simulink model "snap2_f_200msps_64i_4096c"  (R2019a)
settings: Solver=VariableStepDiscrete  StartTime=0.0  StopTime=10.0  RelTol=1e-3
undefined symbols (not defined in the file or in its folder): datetime, posixtime
libraries: xbsIndex_r4 x21354, casper_library_misc x297, casper_library_delays x19, xps_library x14, casper_library_sources x4
(part 60 of 217)

== system snap2_f_200msps_64i_4096c/delay/Subsystem/2 ==
  din : Inport
  delay : Inport  Port=2
  Slice : xbsIndex_r4/Slice  nbits=10  boolean_output=off  mode=Lower Bit Location + Width  bit1=0  base1=MSB of Input  bit0=0  base0=LSB of Input  dbl_ovrd=off  block_type=slice
  Slice1 : xbsIndex_r4/Slice  nbits=2  boolean_output=off  mode=Lower Bit Location + Width  bit1=0  base1=MSB of Input  bit0=10  base0=LSB of Input  dbl_ovrd=off  block_type=slice
  Subsystem1 : Subsystem
  delay_bram_prog_dp : Subsystem  AncestorBlock=casper_library_delays/delay_bram_prog_dp  mask(delay_bram_prog_dp){ram_bits=max_delay_bits-2, bram_latency=2, async=off}
      mask prompts: ram_bits "Max delay (2^?)"; bram_latency "BRAM latency"; async "asynchronous operation"
      mask init:
      | delay_bram_prog_dp_init(gcb, ...
      |     'ram_bits', ram_bits, ...
      |     'bram_latency', bram_latency, ...
      |     'async', async);
  dout : Outport
  wires:
  din/1 -> delay_bram_prog_dp/1(din)
  delay/1 -> Slice1/1, Slice/1
  Slice/1 -> delay_bram_prog_dp/2(delay)
  Slice1/1 -> Subsystem1/2(delay)
  delay_bram_prog_dp/1(dout) -> Subsystem1/1(din)
  Subsystem1/1(dout) -> dout/1

== system snap2_f_200msps_64i_4096c/delay/Subsystem/20 ==
  din : Inport
  delay : Inport  Port=2
  Slice : xbsIndex_r4/Slice  nbits=10  boolean_output=off  mode=Lower Bit Location + Width  bit1=0  base1=MSB of Input  bit0=0  base0=LSB of Input  dbl_ovrd=off  block_type=slice
  Slice1 : xbsIndex_r4/Slice  nbits=2  boolean_output=off  mode=Lower Bit Location + Width  bit1=0  base1=MSB of Input  bit0=10  base0=LSB of Input  dbl_ovrd=off  block_type=slice
  Subsystem1 : Subsystem
  delay_bram_prog_dp : Subsystem  AncestorBlock=casper_library_delays/delay_bram_prog_dp  mask(delay_bram_prog_dp){ram_bits=max_delay_bits-2, bram_latency=2, async=off}
      mask prompts: ram_bits "Max delay (2^?)"; bram_latency "BRAM latency"; async "asynchronous operation"
      mask init:
      | delay_bram_prog_dp_init(gcb, ...
      |     'ram_bits', ram_bits, ...
      |     'bram_latency', bram_latency, ...
      |     'async', async);
  dout : Outport
  wires:
  Subsystem1/1(dout) -> dout/1
  delay_bram_prog_dp/1(dout) -> Subsystem1/1(din)
  Slice1/1 -> Subsystem1/2(delay)
  Slice/1 -> delay_bram_prog_dp/2(delay)
  delay/1 -> Slice/1, Slice1/1
  din/1 -> delay_bram_prog_dp/1(din)

== system snap2_f_200msps_64i_4096c/delay/Subsystem/21 ==
  din : Inport
  delay : Inport  Port=2
  Slice : xbsIndex_r4/Slice  nbits=10  boolean_output=off  mode=Lower Bit Location + Width  bit1=0  base1=MSB of Input  bit0=0  base0=LSB of Input  dbl_ovrd=off  block_type=slice
  Slice1 : xbsIndex_r4/Slice  nbits=2  boolean_output=off  mode=Lower Bit Location + Width  bit1=0  base1=MSB of Input  bit0=10  base0=LSB of Input  dbl_ovrd=off  block_type=slice
  Subsystem1 : Subsystem
  delay_bram_prog_dp : Subsystem  AncestorBlock=casper_library_delays/delay_bram_prog_dp  mask(delay_bram_prog_dp){ram_bits=max_delay_bits-2, bram_latency=2, async=off}
      mask prompts: ram_bits "Max delay (2^?)"; bram_latency "BRAM latency"; async "asynchronous operation"
      mask init:
      | delay_bram_prog_dp_init(gcb, ...
      |     'ram_bits', ram_bits, ...
      |     'bram_latency', bram_latency, ...
      |     'async', async);
  dout : Outport
  wires:
  din/1 -> delay_bram_prog_dp/1(din)
  delay/1 -> Slice1/1, Slice/1
  Slice/1 -> delay_bram_prog_dp/2(delay)
  Slice1/1 -> Subsystem1/2(delay)
  delay_bram_prog_dp/1(dout) -> Subsystem1/1(din)
  Subsystem1/1(dout) -> dout/1

== system snap2_f_200msps_64i_4096c/delay/Subsystem/22 ==
  din : Inport
  delay : Inport  Port=2
  Slice : xbsIndex_r4/Slice  nbits=10  boolean_output=off  mode=Lower Bit Location + Width  bit1=0  base1=MSB of Input  bit0=0  base0=LSB of Input  dbl_ovrd=off  block_type=slice
  Slice1 : xbsIndex_r4/Slice  nbits=2  boolean_output=off  mode=Lower Bit Location + Width  bit1=0  base1=MSB of Input  bit0=10  base0=LSB of Input  dbl_ovrd=off  block_type=slice
  Subsystem1 : Subsystem
  delay_bram_prog_dp : Subsystem  AncestorBlock=casper_library_delays/delay_bram_prog_dp  mask(delay_bram_prog_dp){ram_bits=max_delay_bits-2, bram_latency=2, async=off}
      mask prompts: ram_bits "Max delay (2^?)"; bram_latency "BRAM latency"; async "asynchronous operation"
      mask init:
      | delay_bram_prog_dp_init(gcb, ...
      |     'ram_bits', ram_bits, ...
      |     'bram_latency', bram_latency, ...
      |     'async', async);
  dout : Outport
  wires:
  Subsystem1/1(dout) -> dout/1
  delay_bram_prog_dp/1(dout) -> Subsystem1/1(din)
  Slice1/1 -> Subsystem1/2(delay)
  Slice/1 -> delay_bram_prog_dp/2(delay)
  delay/1 -> Slice/1, Slice1/1
  din/1 -> delay_bram_prog_dp/1(din)

== system snap2_f_200msps_64i_4096c/delay/Subsystem/23 ==
  din : Inport
  delay : Inport  Port=2
  Slice : xbsIndex_r4/Slice  nbits=10  boolean_output=off  mode=Lower Bit Location + Width  bit1=0  base1=MSB of Input  bit0=0  base0=LSB of Input  dbl_ovrd=off  block_type=slice
  Slice1 : xbsIndex_r4/Slice  nbits=2  boolean_output=off  mode=Lower Bit Location + Width  bit1=0  base1=MSB of Input  bit0=10  base0=LSB of Input  dbl_ovrd=off  block_type=slice
  Subsystem1 : Subsystem
  delay_bram_prog_dp : Subsystem  AncestorBlock=casper_library_delays/delay_bram_prog_dp  mask(delay_bram_prog_dp){ram_bits=max_delay_bits-2, bram_latency=2, async=off}
      mask prompts: ram_bits "Max delay (2^?)"; bram_latency "BRAM latency"; async "asynchronous operation"
      mask init:
      | delay_bram_prog_dp_init(gcb, ...
      |     'ram_bits', ram_bits, ...
      |     'bram_latency', bram_latency, ...
      |     'async', async);
  dout : Outport
  wires:
  din/1 -> delay_bram_prog_dp/1(din)
  delay/1 -> Slice1/1, Slice/1
  Slice/1 -> delay_bram_prog_dp/2(delay)
  Slice1/1 -> Subsystem1/2(delay)
  delay_bram_prog_dp/1(dout) -> Subsystem1/1(din)
  Subsystem1/1(dout) -> dout/1

== system snap2_f_200msps_64i_4096c/delay/Subsystem/24 ==
  din : Inport
  delay : Inport  Port=2
  Slice : xbsIndex_r4/Slice  nbits=10  boolean_output=off  mode=Lower Bit Location + Width  bit1=0  base1=MSB of Input  bit0=0  base0=LSB of Input  dbl_ovrd=off  block_type=slice
  Slice1 : xbsIndex_r4/Slice  nbits=2  boolean_output=off  mode=Lower Bit Location + Width  bit1=0  base1=MSB of Input  bit0=10  base0=LSB of Input  dbl_ovrd=off  block_type=slice
  Subsystem1 : Subsystem
  delay_bram_prog_dp : Subsystem  AncestorBlock=casper_library_delays/delay_bram_prog_dp  mask(delay_bram_prog_dp){ram_bits=max_delay_bits-2, bram_latency=2, async=off}
      mask prompts: ram_bits "Max delay (2^?)"; bram_latency "BRAM latency"; async "asynchronous operation"
      mask init:
      | delay_bram_prog_dp_init(gcb, ...
      |     'ram_bits', ram_bits, ...
      |     'bram_latency', bram_latency, ...
      |     'async', async);
  dout : Outport
  wires:
  Subsystem1/1(dout) -> dout/1
  delay_bram_prog_dp/1(dout) -> Subsystem1/1(din)
  Slice1/1 -> Subsystem1/2(delay)
  Slice/1 -> delay_bram_prog_dp/2(delay)
  delay/1 -> Slice/1, Slice1/1
  din/1 -> delay_bram_prog_dp/1(din)

== system snap2_f_200msps_64i_4096c/delay/Subsystem/25 ==
  din : Inport
  delay : Inport  Port=2
  Slice : xbsIndex_r4/Slice  nbits=10  boolean_output=off  mode=Lower Bit Location + Width  bit1=0  base1=MSB of Input  bit0=0  base0=LSB of Input  dbl_ovrd=off  block_type=slice
  Slice1 : xbsIndex_r4/Slice  nbits=2  boolean_output=off  mode=Lower Bit Location + Width  bit1=0  base1=MSB of Input  bit0=10  base0=LSB of Input  dbl_ovrd=off  block_type=slice
  Subsystem1 : Subsystem
  delay_bram_prog_dp : Subsystem  AncestorBlock=casper_library_delays/delay_bram_prog_dp  mask(delay_bram_prog_dp){ram_bits=max_delay_bits-2, bram_latency=2, async=off}
      mask prompts: ram_bits "Max delay (2^?)"; bram_latency "BRAM latency"; async "asynchronous operation"
      mask init:
      | delay_bram_prog_dp_init(gcb, ...
      |     'ram_bits', ram_bits, ...
      |     'bram_latency', bram_latency, ...
      |     'async', async);
  dout : Outport
  wires:
  din/1 -> delay_bram_prog_dp/1(din)
  delay/1 -> Slice1/1, Slice/1
  Slice/1 -> delay_bram_prog_dp/2(delay)
  Slice1/1 -> Subsystem1/2(delay)
  delay_bram_prog_dp/1(dout) -> Subsystem1/1(din)
  Subsystem1/1(dout) -> dout/1

== system snap2_f_200msps_64i_4096c/delay/Subsystem/26 ==
  din : Inport
  delay : Inport  Port=2
  Slice : xbsIndex_r4/Slice  nbits=10  boolean_output=off  mode=Lower Bit Location + Width  bit1=0  base1=MSB of Input  bit0=0  base0=LSB of Input  dbl_ovrd=off  block_type=slice
  Slice1 : xbsIndex_r4/Slice  nbits=2  boolean_output=off  mode=Lower Bit Location + Width  bit1=0  base1=MSB of Input  bit0=10  base0=LSB of Input  dbl_ovrd=off  block_type=slice
  Subsystem1 : Subsystem
  delay_bram_prog_dp : Subsystem  AncestorBlock=casper_library_delays/delay_bram_prog_dp  mask(delay_bram_prog_dp){ram_bits=max_delay_bits-2, bram_latency=2, async=off}
      mask prompts: ram_bits "Max delay (2^?)"; bram_latency "BRAM latency"; async "asynchronous operation"
      mask init:
      | delay_bram_prog_dp_init(gcb, ...
      |     'ram_bits', ram_bits, ...
      |     'bram_latency', bram_latency, ...
      |     'async', async);
  dout : Outport
  wires:
  Subsystem1/1(dout) -> dout/1
  delay_bram_prog_dp/1(dout) -> Subsystem1/1(din)
  Slice1/1 -> Subsystem1/2(delay)
  Slice/1 -> delay_bram_prog_dp/2(delay)
  delay/1 -> Slice/1, Slice1/1
  din/1 -> delay_bram_prog_dp/1(din)

== system snap2_f_200msps_64i_4096c/delay/Subsystem/27 ==
  din : Inport
  delay : Inport  Port=2
  Slice : xbsIndex_r4/Slice  nbits=10  boolean_output=off  mode=Lower Bit Location + Width  bit1=0  base1=MSB of Input  bit0=0  base0=LSB of Input  dbl_ovrd=off  block_type=slice
  Slice1 : xbsIndex_r4/Slice  nbits=2  boolean_output=off  mode=Lower Bit Location + Width  bit1=0  base1=MSB of Input  bit0=10  base0=LSB of Input  dbl_ovrd=off  block_type=slice
  Subsystem1 : Subsystem
  delay_bram_prog_dp : Subsystem  AncestorBlock=casper_library_delays/delay_bram_prog_dp  mask(delay_bram_prog_dp){ram_bits=max_delay_bits-2, bram_latency=2, async=off}
      mask prompts: ram_bits "Max delay (2^?)"; bram_latency "BRAM latency"; async "asynchronous operation"
      mask init:
      | delay_bram_prog_dp_init(gcb, ...
      |     'ram_bits', ram_bits, ...
      |     'bram_latency', bram_latency, ...
      |     'async', async);
  dout : Outport
  wires:
  din/1 -> delay_bram_prog_dp/1(din)
  delay/1 -> Slice1/1, Slice/1
  Slice/1 -> delay_bram_prog_dp/2(delay)
  Slice1/1 -> Subsystem1/2(delay)
  delay_bram_prog_dp/1(dout) -> Subsystem1/1(din)
  Subsystem1/1(dout) -> dout/1

== system snap2_f_200msps_64i_4096c/delay/Subsystem/28 ==
  din : Inport
  delay : Inport  Port=2
  Slice : xbsIndex_r4/Slice  nbits=10  boolean_output=off  mode=Lower Bit Location + Width  bit1=0  base1=MSB of Input  bit0=0  base0=LSB of Input  dbl_ovrd=off  block_type=slice
  Slice1 : xbsIndex_r4/Slice  nbits=2  boolean_output=off  mode=Lower Bit Location + Width  bit1=0  base1=MSB of Input  bit0=10  base0=LSB of Input  dbl_ovrd=off  block_type=slice
  Subsystem1 : Subsystem
  delay_bram_prog_dp : Subsystem  AncestorBlock=casper_library_delays/delay_bram_prog_dp  mask(delay_bram_prog_dp){ram_bits=max_delay_bits-2, bram_latency=2, async=off}
      mask prompts: ram_bits "Max delay (2^?)"; bram_latency "BRAM latency"; async "asynchronous operation"
      mask init:
      | delay_bram_prog_dp_init(gcb, ...
      |     'ram_bits', ram_bits, ...
      |     'bram_latency', bram_latency, ...
      |     'async', async);
  dout : Outport
  wires:
  din/1 -> delay_bram_prog_dp/1(din)
  delay/1 -> Slice1/1, Slice/1
  Slice/1 -> delay_bram_prog_dp/2(delay)
  Slice1/1 -> Subsystem1/2(delay)
  delay_bram_prog_dp/1(dout) -> Subsystem1/1(din)
  Subsystem1/1(dout) -> dout/1

== system snap2_f_200msps_64i_4096c/delay/Subsystem/29 ==
  din : Inport
  delay : Inport  Port=2
  Slice : xbsIndex_r4/Slice  nbits=10  boolean_output=off  mode=Lower Bit Location + Width  bit1=0  base1=MSB of Input  bit0=0  base0=LSB of Input  dbl_ovrd=off  block_type=slice
  Slice1 : xbsIndex_r4/Slice  nbits=2  boolean_output=off  mode=Lower Bit Location + Width  bit1=0  base1=MSB of Input  bit0=10  base0=LSB of Input  dbl_ovrd=off  block_type=slice
  Subsystem1 : Subsystem
  delay_bram_prog_dp : Subsystem  AncestorBlock=casper_library_delays/delay_bram_prog_dp  mask(delay_bram_prog_dp){ram_bits=max_delay_bits-2, bram_latency=2, async=off}
      mask prompts: ram_bits "Max delay (2^?)"; bram_latency "BRAM latency"; async "asynchronous operation"
      mask init:
      | delay_bram_prog_dp_init(gcb, ...
      |     'ram_bits', ram_bits, ...
      |     'bram_latency', bram_latency, ...
      |     'async', async);
  dout : Outport
  wires:
  Subsystem1/1(dout) -> dout/1
  delay_bram_prog_dp/1(dout) -> Subsystem1/1(din)
  Slice1/1 -> Subsystem1/2(delay)
  Slice/1 -> delay_bram_prog_dp/2(delay)
  delay/1 -> Slice/1, Slice1/1
  din/1 -> delay_bram_prog_dp/1(din)

== system snap2_f_200msps_64i_4096c/delay/Subsystem/3 ==
  din : Inport
  delay : Inport  Port=2
  Slice : xbsIndex_r4/Slice  nbits=10  boolean_output=off  mode=Lower Bit Location + Width  bit1=0  base1=MSB of Input  bit0=0  base0=LSB of Input  dbl_ovrd=off  block_type=slice
  Slice1 : xbsIndex_r4/Slice  nbits=2  boolean_output=off  mode=Lower Bit Location + Width  bit1=0  base1=MSB of Input  bit0=10  base0=LSB of Input  dbl_ovrd=off  block_type=slice
  Subsystem1 : Subsystem
  delay_bram_prog_dp : Subsystem  AncestorBlock=casper_library_delays/delay_bram_prog_dp  mask(delay_bram_prog_dp){ram_bits=max_delay_bits-2, bram_latency=2, async=off}
      mask prompts: ram_bits "Max delay (2^?)"; bram_latency "BRAM latency"; async "asynchronous operation"
      mask init:
      | delay_bram_prog_dp_init(gcb, ...
      |     'ram_bits', ram_bits, ...
      |     'bram_latency', bram_latency, ...
      |     'async', async);
  dout : Outport
  wires:
  Subsystem1/1(dout) -> dout/1
  delay_bram_prog_dp/1(dout) -> Subsystem1/1(din)
  Slice1/1 -> Subsystem1/2(delay)
  Slice/1 -> delay_bram_prog_dp/2(delay)
  delay/1 -> Slice/1, Slice1/1
  din/1 -> delay_bram_prog_dp/1(din)

== system snap2_f_200msps_64i_4096c/delay/Subsystem/30 ==
  din : Inport
  delay : Inport  Port=2
  Slice : xbsIndex_r4/Slice  nbits=10  boolean_output=off  mode=Lower Bit Location + Width  bit1=0  base1=MSB of Input  bit0=0  base0=LSB of Input  dbl_ovrd=off  block_type=slice
  Slice1 : xbsIndex_r4/Slice  nbits=2  boolean_output=off  mode=Lower Bit Location + Width  bit1=0  base1=MSB of Input  bit0=10  base0=LSB of Input  dbl_ovrd=off  block_type=slice
  Subsystem1 : Subsystem
  delay_bram_prog_dp : Subsystem  AncestorBlock=casper_library_delays/delay_bram_prog_dp  mask(delay_bram_prog_dp){ram_bits=max_delay_bits-2, bram_latency=2, async=off}
      mask prompts: ram_bits "Max delay (2^?)"; bram_latency "BRAM latency"; async "asynchronous operation"
      mask init:
      | delay_bram_prog_dp_init(gcb, ...
      |     'ram_bits', ram_bits, ...
      |     'bram_latency', bram_latency, ...
      |     'async', async);
  dout : Outport
  wires:
  din/1 -> delay_bram_prog_dp/1(din)
  delay/1 -> Slice1/1, Slice/1
  Slice/1 -> delay_bram_prog_dp/2(delay)
  Slice1/1 -> Subsystem1/2(delay)
  delay_bram_prog_dp/1(dout) -> Subsystem1/1(din)
  Subsystem1/1(dout) -> dout/1

== system snap2_f_200msps_64i_4096c/delay/Subsystem/31 ==
  din : Inport
  delay : Inport  Port=2
  Slice : xbsIndex_r4/Slice  nbits=10  boolean_output=off  mode=Lower Bit Location + Width  bit1=0  base1=MSB of Input  bit0=0  base0=LSB of Input  dbl_ovrd=off  block_type=slice
  Slice1 : xbsIndex_r4/Slice  nbits=2  boolean_output=off  mode=Lower Bit Location + Width  bit1=0  base1=MSB of Input  bit0=10  base0=LSB of Input  dbl_ovrd=off  block_type=slice
  Subsystem1 : Subsystem
  delay_bram_prog_dp : Subsystem  AncestorBlock=casper_library_delays/delay_bram_prog_dp  mask(delay_bram_prog_dp){ram_bits=max_delay_bits-2, bram_latency=2, async=off}
      mask prompts: ram_bits "Max delay (2^?)"; bram_latency "BRAM latency"; async "asynchronous operation"
      mask init:
      | delay_bram_prog_dp_init(gcb, ...
      |     'ram_bits', ram_bits, ...
      |     'bram_latency', bram_latency, ...
      |     'async', async);
  dout : Outport
  wires:
  Subsystem1/1(dout) -> dout/1
  delay_bram_prog_dp/1(dout) -> Subsystem1/1(din)
  Slice1/1 -> Subsystem1/2(delay)
  Slice/1 -> delay_bram_prog_dp/2(delay)
  delay/1 -> Slice/1, Slice1/1
  din/1 -> delay_bram_prog_dp/1(din)

== system snap2_f_200msps_64i_4096c/delay/Subsystem/32 ==
  din : Inport
  delay : Inport  Port=2
  Slice : xbsIndex_r4/Slice  nbits=10  boolean_output=off  mode=Lower Bit Location + Width  bit1=0  base1=MSB of Input  bit0=0  base0=LSB of Input  dbl_ovrd=off  block_type=slice
  Slice1 : xbsIndex_r4/Slice  nbits=2  boolean_output=off  mode=Lower Bit Location + Width  bit1=0  base1=MSB of Input  bit0=10  base0=LSB of Input  dbl_ovrd=off  block_type=slice
  Subsystem1 : Subsystem
  delay_bram_prog_dp : Subsystem  AncestorBlock=casper_library_delays/delay_bram_prog_dp  mask(delay_bram_prog_dp){ram_bits=max_delay_bits-2, bram_latency=2, async=off}
      mask prompts: ram_bits "Max delay (2^?)"; bram_latency "BRAM latency"; async "asynchronous operation"
      mask init:
      | delay_bram_prog_dp_init(gcb, ...
      |     'ram_bits', ram_bits, ...
      |     'bram_latency', bram_latency, ...
      |     'async', async);
  dout : Outport
  wires:
  din/1 -> delay_bram_prog_dp/1(din)
  delay/1 -> Slice1/1, Slice/1
  Slice/1 -> delay_bram_prog_dp/2(delay)
  Slice1/1 -> Subsystem1/2(delay)
  delay_bram_prog_dp/1(dout) -> Subsystem1/1(din)
  Subsystem1/1(dout) -> dout/1

== system snap2_f_200msps_64i_4096c/delay/Subsystem/33 ==
  din : Inport
  delay : Inport  Port=2
  Slice : xbsIndex_r4/Slice  nbits=10  boolean_output=off  mode=Lower Bit Location + Width  bit1=0  base1=MSB of Input  bit0=0  base0=LSB of Input  dbl_ovrd=off  block_type=slice
  Slice1 : xbsIndex_r4/Slice  nbits=2  boolean_output=off  mode=Lower Bit Location + Width  bit1=0  base1=MSB of Input  bit0=10  base0=LSB of Input  dbl_ovrd=off  block_type=slice
  Subsystem1 : Subsystem
  delay_bram_prog_dp : Subsystem  AncestorBlock=casper_library_delays/delay_bram_prog_dp  mask(delay_bram_prog_dp){ram_bits=max_delay_bits-2, bram_latency=2, async=off}
      mask prompts: ram_bits "Max delay (2^?)"; bram_latency "BRAM latency"; async "asynchronous operation"
      mask init:
      | delay_bram_prog_dp_init(gcb, ...
      |     'ram_bits', ram_bits, ...
      |     'bram_latency', bram_latency, ...
      |     'async', async);
  dout : Outport
  wires:
  Subsystem1/1(dout) -> dout/1
  delay_bram_prog_dp/1(dout) -> Subsystem1/1(din)
  Slice1/1 -> Subsystem1/2(delay)
  Slice/1 -> delay_bram_prog_dp/2(delay)
  delay/1 -> Slice/1, Slice1/1
  din/1 -> delay_bram_prog_dp/1(din)

== system snap2_f_200msps_64i_4096c/delay/Subsystem/34 ==
  din : Inport
  delay : Inport  Port=2
  Slice : xbsIndex_r4/Slice  nbits=10  boolean_output=off  mode=Lower Bit Location + Width  bit1=0  base1=MSB of Input  bit0=0  base0=LSB of Input  dbl_ovrd=off  block_type=slice
  Slice1 : xbsIndex_r4/Slice  nbits=2  boolean_output=off  mode=Lower Bit Location + Width  bit1=0  base1=MSB of Input  bit0=10  base0=LSB of Input  dbl_ovrd=off  block_type=slice
  Subsystem1 : Subsystem
  delay_bram_prog_dp : Subsystem  AncestorBlock=casper_library_delays/delay_bram_prog_dp  mask(delay_bram_prog_dp){ram_bits=max_delay_bits-2, bram_latency=2, async=off}
      mask prompts: ram_bits "Max delay (2^?)"; bram_latency "BRAM latency"; async "asynchronous operation"
      mask init:
      | delay_bram_prog_dp_init(gcb, ...
      |     'ram_bits', ram_bits, ...
      |     'bram_latency', bram_latency, ...
      |     'async', async);
  dout : Outport
  wires:
  din/1 -> delay_bram_prog_dp/1(din)
  delay/1 -> Slice1/1, Slice/1
  Slice/1 -> delay_bram_prog_dp/2(delay)
  Slice1/1 -> Subsystem1/2(delay)
  delay_bram_prog_dp/1(dout) -> Subsystem1/1(din)
  Subsystem1/1(dout) -> dout/1

== system snap2_f_200msps_64i_4096c/delay/Subsystem/35 ==
  din : Inport
  delay : Inport  Port=2
  Slice : xbsIndex_r4/Slice  nbits=10  boolean_output=off  mode=Lower Bit Location + Width  bit1=0  base1=MSB of Input  bit0=0  base0=LSB of Input  dbl_ovrd=off  block_type=slice
  Slice1 : xbsIndex_r4/Slice  nbits=2  boolean_output=off  mode=Lower Bit Location + Width  bit1=0  base1=MSB of Input  bit0=10  base0=LSB of Input  dbl_ovrd=off  block_type=slice
  Subsystem1 : Subsystem
  delay_bram_prog_dp : Subsystem  AncestorBlock=casper_library_delays/delay_bram_prog_dp  mask(delay_bram_prog_dp){ram_bits=max_delay_bits-2, bram_latency=2, async=off}
      mask prompts: ram_bits "Max delay (2^?)"; bram_latency "BRAM latency"; async "asynchronous operation"
      mask init:
      | delay_bram_prog_dp_init(gcb, ...
      |     'ram_bits', ram_bits, ...
      |     'bram_latency', bram_latency, ...
      |     'async', async);
  dout : Outport
  wires:
  Subsystem1/1(dout) -> dout/1
  delay_bram_prog_dp/1(dout) -> Subsystem1/1(din)
  Slice1/1 -> Subsystem1/2(delay)
  Slice/1 -> delay_bram_prog_dp/2(delay)
  delay/1 -> Slice/1, Slice1/1
  din/1 -> delay_bram_prog_dp/1(din)

== system snap2_f_200msps_64i_4096c/delay/Subsystem/36 ==
  din : Inport
  delay : Inport  Port=2
  Slice : xbsIndex_r4/Slice  nbits=10  boolean_output=off  mode=Lower Bit Location + Width  bit1=0  base1=MSB of Input  bit0=0  base0=LSB of Input  dbl_ovrd=off  block_type=slice
  Slice1 : xbsIndex_r4/Slice  nbits=2  boolean_output=off  mode=Lower Bit Location + Width  bit1=0  base1=MSB of Input  bit0=10  base0=LSB of Input  dbl_ovrd=off  block_type=slice
  Subsystem1 : Subsystem
  delay_bram_prog_dp : Subsystem  AncestorBlock=casper_library_delays/delay_bram_prog_dp  mask(delay_bram_prog_dp){ram_bits=max_delay_bits-2, bram_latency=2, async=off}
      mask prompts: ram_bits "Max delay (2^?)"; bram_latency "BRAM latency"; async "asynchronous operation"
      mask init:
      | delay_bram_prog_dp_init(gcb, ...
      |     'ram_bits', ram_bits, ...
      |     'bram_latency', bram_latency, ...
      |     'async', async);
  dout : Outport
  wires:
  Subsystem1/1(dout) -> dout/1
  delay_bram_prog_dp/1(dout) -> Subsystem1/1(din)
  Slice1/1 -> Subsystem1/2(delay)
  Slice/1 -> delay_bram_prog_dp/2(delay)
  delay/1 -> Slice/1, Slice1/1
  din/1 -> delay_bram_prog_dp/1(din)

== system snap2_f_200msps_64i_4096c/delay/Subsystem/37 ==
  din : Inport
  delay : Inport  Port=2
  Slice : xbsIndex_r4/Slice  nbits=10  boolean_output=off  mode=Lower Bit Location + Width  bit1=0  base1=MSB of Input  bit0=0  base0=LSB of Input  dbl_ovrd=off  block_type=slice
  Slice1 : xbsIndex_r4/Slice  nbits=2  boolean_output=off  mode=Lower Bit Location + Width  bit1=0  base1=MSB of Input  bit0=10  base0=LSB of Input  dbl_ovrd=off  block_type=slice
  Subsystem1 : Subsystem
  delay_bram_prog_dp : Subsystem  AncestorBlock=casper_library_delays/delay_bram_prog_dp  mask(delay_bram_prog_dp){ram_bits=max_delay_bits-2, bram_latency=2, async=off}
      mask prompts: ram_bits "Max delay (2^?)"; bram_latency "BRAM latency"; async "asynchronous operation"
      mask init:
      | delay_bram_prog_dp_init(gcb, ...
      |     'ram_bits', ram_bits, ...
      |     'bram_latency', bram_latency, ...
      |     'async', async);
  dout : Outport
  wires:
  din/1 -> delay_bram_prog_dp/1(din)
  delay/1 -> Slice1/1, Slice/1
  Slice/1 -> delay_bram_prog_dp/2(delay)
  Slice1/1 -> Subsystem1/2(delay)
  delay_bram_prog_dp/1(dout) -> Subsystem1/1(din)
  Subsystem1/1(dout) -> dout/1

== system snap2_f_200msps_64i_4096c/delay/Subsystem/38 ==
  din : Inport
  delay : Inport  Port=2
  Slice : xbsIndex_r4/Slice  nbits=10  boolean_output=off  mode=Lower Bit Location + Width  bit1=0  base1=MSB of Input  bit0=0  base0=LSB of Input  dbl_ovrd=off  block_type=slice
  Slice1 : xbsIndex_r4/Slice  nbits=2  boolean_output=off  mode=Lower Bit Location + Width  bit1=0  base1=MSB of Input  bit0=10  base0=LSB of Input  dbl_ovrd=off  block_type=slice
  Subsystem1 : Subsystem
  delay_bram_prog_dp : Subsystem  AncestorBlock=casper_library_delays/delay_bram_prog_dp  mask(delay_bram_prog_dp){ram_bits=max_delay_bits-2, bram_latency=2, async=off}
      mask prompts: ram_bits "Max delay (2^?)"; bram_latency "BRAM latency"; async "asynchronous operation"
      mask init:
      | delay_bram_prog_dp_init(gcb, ...
      |     'ram_bits', ram_bits, ...
      |     'bram_latency', bram_latency, ...
      |     'async', async);
  dout : Outport
  wires:
  Subsystem1/1(dout) -> dout/1
  delay_bram_prog_dp/1(dout) -> Subsystem1/1(din)
  Slice1/1 -> Subsystem1/2(delay)
  Slice/1 -> delay_bram_prog_dp/2(delay)
  delay/1 -> Slice/1, Slice1/1
  din/1 -> delay_bram_prog_dp/1(din)

== system snap2_f_200msps_64i_4096c/delay/Subsystem/39 ==
  din : Inport
  delay : Inport  Port=2
  Slice : xbsIndex_r4/Slice  nbits=10  boolean_output=off  mode=Lower Bit Location + Width  bit1=0  base1=MSB of Input  bit0=0  base0=LSB of Input  dbl_ovrd=off  block_type=slice
  Slice1 : xbsIndex_r4/Slice  nbits=2  boolean_output=off  mode=Lower Bit Location + Width  bit1=0  base1=MSB of Input  bit0=10  base0=LSB of Input  dbl_ovrd=off  block_type=slice
  Subsystem1 : Subsystem
  delay_bram_prog_dp : Subsystem  AncestorBlock=casper_library_delays/delay_bram_prog_dp  mask(delay_bram_prog_dp){ram_bits=max_delay_bits-2, bram_latency=2, async=off}
      mask prompts: ram_bits "Max delay (2^?)"; bram_latency "BRAM latency"; async "asynchronous operation"
      mask init:
      | delay_bram_prog_dp_init(gcb, ...
      |     'ram_bits', ram_bits, ...
      |     'bram_latency', bram_latency, ...
      |     'async', async);
  dout : Outport
  wires:
  din/1 -> delay_bram_prog_dp/1(din)
  delay/1 -> Slice1/1, Slice/1
  Slice/1 -> delay_bram_prog_dp/2(delay)
  Slice1/1 -> Subsystem1/2(delay)
  delay_bram_prog_dp/1(dout) -> Subsystem1/1(din)
  Subsystem1/1(dout) -> dout/1

== system snap2_f_200msps_64i_4096c/delay/Subsystem/4 ==
  din : Inport
  delay : Inport  Port=2
  Slice : xbsIndex_r4/Slice  nbits=10  boolean_output=off  mode=Lower Bit Location + Width  bit1=0  base1=MSB of Input  bit0=0  base0=LSB of Input  dbl_ovrd=off  block_type=slice
  Slice1 : xbsIndex_r4/Slice  nbits=2  boolean_output=off  mode=Lower Bit Location + Width  bit1=0  base1=MSB of Input  bit0=10  base0=LSB of Input  dbl_ovrd=off  block_type=slice
  Subsystem1 : Subsystem
  delay_bram_prog_dp : Subsystem  AncestorBlock=casper_library_delays/delay_bram_prog_dp  mask(delay_bram_prog_dp){ram_bits=max_delay_bits-2, bram_latency=2, async=off}
      mask prompts: ram_bits "Max delay (2^?)"; bram_latency "BRAM latency"; async "asynchronous operation"
      mask init:
      | delay_bram_prog_dp_init(gcb, ...
      |     'ram_bits', ram_bits, ...
      |     'bram_latency', bram_latency, ...
      |     'async', async);
  dout : Outport
  wires:
  din/1 -> delay_bram_prog_dp/1(din)
  delay/1 -> Slice1/1, Slice/1
  Slice/1 -> delay_bram_prog_dp/2(delay)
  Slice1/1 -> Subsystem1/2(delay)
  delay_bram_prog_dp/1(dout) -> Subsystem1/1(din)
  Subsystem1/1(dout) -> dout/1

== system snap2_f_200msps_64i_4096c/delay/Subsystem/40 ==
  din : Inport
  delay : Inport  Port=2
  Slice : xbsIndex_r4/Slice  nbits=10  boolean_output=off  mode=Lower Bit Location + Width  bit1=0  base1=MSB of Input  bit0=0  base0=LSB of Input  dbl_ovrd=off  block_type=slice
  Slice1 : xbsIndex_r4/Slice  nbits=2  boolean_output=off  mode=Lower Bit Location + Width  bit1=0  base1=MSB of Input  bit0=10  base0=LSB of Input  dbl_ovrd=off  block_type=slice
  Subsystem1 : Subsystem
  delay_bram_prog_dp : Subsystem  AncestorBlock=casper_library_delays/delay_bram_prog_dp  mask(delay_bram_prog_dp){ram_bits=max_delay_bits-2, bram_latency=2, async=off}
      mask prompts: ram_bits "Max delay (2^?)"; bram_latency "BRAM latency"; async "asynchronous operation"
      mask init:
      | delay_bram_prog_dp_init(gcb, ...
      |     'ram_bits', ram_bits, ...
      |     'bram_latency', bram_latency, ...
      |     'async', async);
  dout : Outport
  wires:
  Subsystem1/1(dout) -> dout/1
  delay_bram_prog_dp/1(dout) -> Subsystem1/1(din)
  Slice1/1 -> Subsystem1/2(delay)
  Slice/1 -> delay_bram_prog_dp/2(delay)
  delay/1 -> Slice/1, Slice1/1
  din/1 -> delay_bram_prog_dp/1(din)

== system snap2_f_200msps_64i_4096c/delay/Subsystem/41 ==
  din : Inport
  delay : Inport  Port=2
  Slice : xbsIndex_r4/Slice  nbits=10  boolean_output=off  mode=Lower Bit Location + Width  bit1=0  base1=MSB of Input  bit0=0  base0=LSB of Input  dbl_ovrd=off  block_type=slice
  Slice1 : xbsIndex_r4/Slice  nbits=2  boolean_output=off  mode=Lower Bit Location + Width  bit1=0  base1=MSB of Input  bit0=10  base0=LSB of Input  dbl_ovrd=off  block_type=slice
  Subsystem1 : Subsystem
  delay_bram_prog_dp : Subsystem  AncestorBlock=casper_library_delays/delay_bram_prog_dp  mask(delay_bram_prog_dp){ram_bits=max_delay_bits-2, bram_latency=2, async=off}
      mask prompts: ram_bits "Max delay (2^?)"; bram_latency "BRAM latency"; async "asynchronous operation"
      mask init:
      | delay_bram_prog_dp_init(gcb, ...
      |     'ram_bits', ram_bits, ...
      |     'bram_latency', bram_latency, ...
      |     'async', async);
  dout : Outport
  wires:
  din/1 -> delay_bram_prog_dp/1(din)
  delay/1 -> Slice1/1, Slice/1
  Slice/1 -> delay_bram_prog_dp/2(delay)
  Slice1/1 -> Subsystem1/2(delay)
  delay_bram_prog_dp/1(dout) -> Subsystem1/1(din)
  Subsystem1/1(dout) -> dout/1

== system snap2_f_200msps_64i_4096c/delay/Subsystem/42 ==
  din : Inport
  delay : Inport  Port=2
  Slice : xbsIndex_r4/Slice  nbits=10  boolean_output=off  mode=Lower Bit Location + Width  bit1=0  base1=MSB of Input  bit0=0  base0=LSB of Input  dbl_ovrd=off  block_type=slice
  Slice1 : xbsIndex_r4/Slice  nbits=2  boolean_output=off  mode=Lower Bit Location + Width  bit1=0  base1=MSB of Input  bit0=10  base0=LSB of Input  dbl_ovrd=off  block_type=slice
  Subsystem1 : Subsystem
  delay_bram_prog_dp : Subsystem  AncestorBlock=casper_library_delays/delay_bram_prog_dp  mask(delay_bram_prog_dp){ram_bits=max_delay_bits-2, bram_latency=2, async=off}
      mask prompts: ram_bits "Max delay (2^?)"; bram_latency "BRAM latency"; async "asynchronous operation"
      mask init:
      | delay_bram_prog_dp_init(gcb, ...
      |     'ram_bits', ram_bits, ...
      |     'bram_latency', bram_latency, ...
      |     'async', async);
  dout : Outport
  wires:
  Subsystem1/1(dout) -> dout/1
  delay_bram_prog_dp/1(dout) -> Subsystem1/1(din)
  Slice1/1 -> Subsystem1/2(delay)
  Slice/1 -> delay_bram_prog_dp/2(delay)
  delay/1 -> Slice/1, Slice1/1
  din/1 -> delay_bram_prog_dp/1(din)

== system snap2_f_200msps_64i_4096c/delay/Subsystem/43 ==
  din : Inport
  delay : Inport  Port=2
  Slice : xbsIndex_r4/Slice  nbits=10  boolean_output=off  mode=Lower Bit Location + Width  bit1=0  base1=MSB of Input  bit0=0  base0=LSB of Input  dbl_ovrd=off  block_type=slice
  Slice1 : xbsIndex_r4/Slice  nbits=2  boolean_output=off  mode=Lower Bit Location + Width  bit1=0  base1=MSB of Input  bit0=10  base0=LSB of Input  dbl_ovrd=off  block_type=slice
  Subsystem1 : Subsystem
  delay_bram_prog_dp : Subsystem  AncestorBlock=casper_library_delays/delay_bram_prog_dp  mask(delay_bram_prog_dp){ram_bits=max_delay_bits-2, bram_latency=2, async=off}
      mask prompts: ram_bits "Max delay (2^?)"; bram_latency "BRAM latency"; async "asynchronous operation"
      mask init:
      | delay_bram_prog_dp_init(gcb, ...
      |     'ram_bits', ram_bits, ...
      |     'bram_latency', bram_latency, ...
      |     'async', async);
  dout : Outport
  wires:
  din/1 -> delay_bram_prog_dp/1(din)
  delay/1 -> Slice1/1, Slice/1
  Slice/1 -> delay_bram_prog_dp/2(delay)
  Slice1/1 -> Subsystem1/2(delay)
  delay_bram_prog_dp/1(dout) -> Subsystem1/1(din)
  Subsystem1/1(dout) -> dout/1

== system snap2_f_200msps_64i_4096c/delay/Subsystem/44 ==
  din : Inport
  delay : Inport  Port=2
  Slice : xbsIndex_r4/Slice  nbits=10  boolean_output=off  mode=Lower Bit Location + Width  bit1=0  base1=MSB of Input  bit0=0  base0=LSB of Input  dbl_ovrd=off  block_type=slice
  Slice1 : xbsIndex_r4/Slice  nbits=2  boolean_output=off  mode=Lower Bit Location + Width  bit1=0  base1=MSB of Input  bit0=10  base0=LSB of Input  dbl_ovrd=off  block_type=slice
  Subsystem1 : Subsystem
  delay_bram_prog_dp : Subsystem  AncestorBlock=casper_library_delays/delay_bram_prog_dp  mask(delay_bram_prog_dp){ram_bits=max_delay_bits-2, bram_latency=2, async=off}
      mask prompts: ram_bits "Max delay (2^?)"; bram_latency "BRAM latency"; async "asynchronous operation"
      mask init:
      | delay_bram_prog_dp_init(gcb, ...
      |     'ram_bits', ram_bits, ...
      |     'bram_latency', bram_latency, ...
      |     'async', async);
  dout : Outport
  wires:
  din/1 -> delay_bram_prog_dp/1(din)
  delay/1 -> Slice1/1, Slice/1
  Slice/1 -> delay_bram_prog_dp/2(delay)
  Slice1/1 -> Subsystem1/2(delay)
  delay_bram_prog_dp/1(dout) -> Subsystem1/1(din)
  Subsystem1/1(dout) -> dout/1

== system snap2_f_200msps_64i_4096c/delay/Subsystem/45 ==
  din : Inport
  delay : Inport  Port=2
  Slice : xbsIndex_r4/Slice  nbits=10  boolean_output=off  mode=Lower Bit Location + Width  bit1=0  base1=MSB of Input  bit0=0  base0=LSB of Input  dbl_ovrd=off  block_type=slice
  Slice1 : xbsIndex_r4/Slice  nbits=2  boolean_output=off  mode=Lower Bit Location + Width  bit1=0  base1=MSB of Input  bit0=10  base0=LSB of Input  dbl_ovrd=off  block_type=slice
  Subsystem1 : Subsystem
  delay_bram_prog_dp : Subsystem  AncestorBlock=casper_library_delays/delay_bram_prog_dp  mask(delay_bram_prog_dp){ram_bits=max_delay_bits-2, bram_latency=2, async=off}
      mask prompts: ram_bits "Max delay (2^?)"; bram_latency "BRAM latency"; async "asynchronous operation"
      mask init:
      | delay_bram_prog_dp_init(gcb, ...
      |     'ram_bits', ram_bits, ...
      |     'bram_latency', bram_latency, ...
      |     'async', async);
  dout : Outport
  wires:
  Subsystem1/1(dout) -> dout/1
  delay_bram_prog_dp/1(dout) -> Subsystem1/1(din)
  Slice1/1 -> Subsystem1/2(delay)
  Slice/1 -> delay_bram_prog_dp/2(delay)
  delay/1 -> Slice/1, Slice1/1
  din/1 -> delay_bram_prog_dp/1(din)

== system snap2_f_200msps_64i_4096c/delay/Subsystem/46 ==
  din : Inport
  delay : Inport  Port=2
  Slice : xbsIndex_r4/Slice  nbits=10  boolean_output=off  mode=Lower Bit Location + Width  bit1=0  base1=MSB of Input  bit0=0  base0=LSB of Input  dbl_ovrd=off  block_type=slice
  Slice1 : xbsIndex_r4/Slice  nbits=2  boolean_output=off  mode=Lower Bit Location + Width  bit1=0  base1=MSB of Input  bit0=10  base0=LSB of Input  dbl_ovrd=off  block_type=slice
  Subsystem1 : Subsystem
  delay_bram_prog_dp : Subsystem  AncestorBlock=casper_library_delays/delay_bram_prog_dp  mask(delay_bram_prog_dp){ram_bits=max_delay_bits-2, bram_latency=2, async=off}
      mask prompts: ram_bits "Max delay (2^?)"; bram_latency "BRAM latency"; async "asynchronous operation"
      mask init:
      | delay_bram_prog_dp_init(gcb, ...
      |     'ram_bits', ram_bits, ...
      |     'bram_latency', bram_latency, ...
      |     'async', async);
  dout : Outport
  wires:
  din/1 -> delay_bram_prog_dp/1(din)
  delay/1 -> Slice1/1, Slice/1
  Slice/1 -> delay_bram_prog_dp/2(delay)
  Slice1/1 -> Subsystem1/2(delay)
  delay_bram_prog_dp/1(dout) -> Subsystem1/1(din)
  Subsystem1/1(dout) -> dout/1

== system snap2_f_200msps_64i_4096c/delay/Subsystem/47 ==
  din : Inport
  delay : Inport  Port=2
  Slice : xbsIndex_r4/Slice  nbits=10  boolean_output=off  mode=Lower Bit Location + Width  bit1=0  base1=MSB of Input  bit0=0  base0=LSB of Input  dbl_ovrd=off  block_type=slice
  Slice1 : xbsIndex_r4/Slice  nbits=2  boolean_output=off  mode=Lower Bit Location + Width  bit1=0  base1=MSB of Input  bit0=10  base0=LSB of Input  dbl_ovrd=off  block_type=slice
  Subsystem1 : Subsystem
  delay_bram_prog_dp : Subsystem  AncestorBlock=casper_library_delays/delay_bram_prog_dp  mask(delay_bram_prog_dp){ram_bits=max_delay_bits-2, bram_latency=2, async=off}
      mask prompts: ram_bits "Max delay (2^?)"; bram_latency "BRAM latency"; async "asynchronous operation"
      mask init:
      | delay_bram_prog_dp_init(gcb, ...
      |     'ram_bits', ram_bits, ...
      |     'bram_latency', bram_latency, ...
      |     'async', async);
  dout : Outport
  wires:
  Subsystem1/1(dout) -> dout/1
  delay_bram_prog_dp/1(dout) -> Subsystem1/1(din)
  Slice1/1 -> Subsystem1/2(delay)
  Slice/1 -> delay_bram_prog_dp/2(delay)
  delay/1 -> Slice/1, Slice1/1
  din/1 -> delay_bram_prog_dp/1(din)

== system snap2_f_200msps_64i_4096c/delay/Subsystem/48 ==
  din : Inport
  delay : Inport  Port=2
  Slice : xbsIndex_r4/Slice  nbits=10  boolean_output=off  mode=Lower Bit Location + Width  bit1=0  base1=MSB of Input  bit0=0  base0=LSB of Input  dbl_ovrd=off  block_type=slice
  Slice1 : xbsIndex_r4/Slice  nbits=2  boolean_output=off  mode=Lower Bit Location + Width  bit1=0  base1=MSB of Input  bit0=10  base0=LSB of Input  dbl_ovrd=off  block_type=slice
  Subsystem1 : Subsystem
  delay_bram_prog_dp : Subsystem  AncestorBlock=casper_library_delays/delay_bram_prog_dp  mask(delay_bram_prog_dp){ram_bits=max_delay_bits-2, bram_latency=2, async=off}
      mask prompts: ram_bits "Max delay (2^?)"; bram_latency "BRAM latency"; async "asynchronous operation"
      mask init:
      | delay_bram_prog_dp_init(gcb, ...
      |     'ram_bits', ram_bits, ...
      |     'bram_latency', bram_latency, ...
      |     'async', async);
  dout : Outport
  wires:
  din/1 -> delay_bram_prog_dp/1(din)
  delay/1 -> Slice1/1, Slice/1
  Slice/1 -> delay_bram_prog_dp/2(delay)
  Slice1/1 -> Subsystem1/2(delay)
  delay_bram_prog_dp/1(dout) -> Subsystem1/1(din)
  Subsystem1/1(dout) -> dout/1

== system snap2_f_200msps_64i_4096c/delay/Subsystem/49 ==
  din : Inport
  delay : Inport  Port=2
  Slice : xbsIndex_r4/Slice  nbits=10  boolean_output=off  mode=Lower Bit Location + Width  bit1=0  base1=MSB of Input  bit0=0  base0=LSB of Input  dbl_ovrd=off  block_type=slice
  Slice1 : xbsIndex_r4/Slice  nbits=2  boolean_output=off  mode=Lower Bit Location + Width  bit1=0  base1=MSB of Input  bit0=10  base0=LSB of Input  dbl_ovrd=off  block_type=slice
  Subsystem1 : Subsystem
  delay_bram_prog_dp : Subsystem  AncestorBlock=casper_library_delays/delay_bram_prog_dp  mask(delay_bram_prog_dp){ram_bits=max_delay_bits-2, bram_latency=2, async=off}
      mask prompts: ram_bits "Max delay (2^?)"; bram_latency "BRAM latency"; async "asynchronous operation"
      mask init:
      | delay_bram_prog_dp_init(gcb, ...
      |     'ram_bits', ram_bits, ...
      |     'bram_latency', bram_latency, ...
      |     'async', async);
  dout : Outport
  wires:
  Subsystem1/1(dout) -> dout/1
  delay_bram_prog_dp/1(dout) -> Subsystem1/1(din)
  Slice1/1 -> Subsystem1/2(delay)
  Slice/1 -> delay_bram_prog_dp/2(delay)
  delay/1 -> Slice/1, Slice1/1
  din/1 -> delay_bram_prog_dp/1(din)

== system snap2_f_200msps_64i_4096c/delay/Subsystem/5 ==
  din : Inport
  delay : Inport  Port=2
  Slice : xbsIndex_r4/Slice  nbits=10  boolean_output=off  mode=Lower Bit Location + Width  bit1=0  base1=MSB of Input  bit0=0  base0=LSB of Input  dbl_ovrd=off  block_type=slice
  Slice1 : xbsIndex_r4/Slice  nbits=2  boolean_output=off  mode=Lower Bit Location + Width  bit1=0  base1=MSB of Input  bit0=10  base0=LSB of Input  dbl_ovrd=off  block_type=slice
  Subsystem1 : Subsystem
  delay_bram_prog_dp : Subsystem  AncestorBlock=casper_library_delays/delay_bram_prog_dp  mask(delay_bram_prog_dp){ram_bits=max_delay_bits-2, bram_latency=2, async=off}
      mask prompts: ram_bits "Max delay (2^?)"; bram_latency "BRAM latency"; async "asynchronous operation"
      mask init:
      | delay_bram_prog_dp_init(gcb, ...
      |     'ram_bits', ram_bits, ...
      |     'bram_latency', bram_latency, ...
      |     'async', async);
  dout : Outport
  wires:
  Subsystem1/1(dout) -> dout/1
  delay_bram_prog_dp/1(dout) -> Subsystem1/1(din)
  Slice1/1 -> Subsystem1/2(delay)
  Slice/1 -> delay_bram_prog_dp/2(delay)
  delay/1 -> Slice/1, Slice1/1
  din/1 -> delay_bram_prog_dp/1(din)

== system snap2_f_200msps_64i_4096c/delay/Subsystem/50 ==
  din : Inport
  delay : Inport  Port=2
  Slice : xbsIndex_r4/Slice  nbits=10  boolean_output=off  mode=Lower Bit Location + Width  bit1=0  base1=MSB of Input  bit0=0  base0=LSB of Input  dbl_ovrd=off  block_type=slice
  Slice1 : xbsIndex_r4/Slice  nbits=2  boolean_output=off  mode=Lower Bit Location + Width  bit1=0  base1=MSB of Input  bit0=10  base0=LSB of Input  dbl_ovrd=off  block_type=slice
  Subsystem1 : Subsystem
  delay_bram_prog_dp : Subsystem  AncestorBlock=casper_library_delays/delay_bram_prog_dp  mask(delay_bram_prog_dp){ram_bits=max_delay_bits-2, bram_latency=2, async=off}
      mask prompts: ram_bits "Max delay (2^?)"; bram_latency "BRAM latency"; async "asynchronous operation"
      mask init:
      | delay_bram_prog_dp_init(gcb, ...
      |     'ram_bits', ram_bits, ...
      |     'bram_latency', bram_latency, ...
      |     'async', async);
  dout : Outport
  wires:
  din/1 -> delay_bram_prog_dp/1(din)
  delay/1 -> Slice1/1, Slice/1
  Slice/1 -> delay_bram_prog_dp/2(delay)
  Slice1/1 -> Subsystem1/2(delay)
  delay_bram_prog_dp/1(dout) -> Subsystem1/1(din)
  Subsystem1/1(dout) -> dout/1

== system snap2_f_200msps_64i_4096c/delay/Subsystem/51 ==
  din : Inport
  delay : Inport  Port=2
  Slice : xbsIndex_r4/Slice  nbits=10  boolean_output=off  mode=Lower Bit Location + Width  bit1=0  base1=MSB of Input  bit0=0  base0=LSB of Input  dbl_ovrd=off  block_type=slice
  Slice1 : xbsIndex_r4/Slice  nbits=2  boolean_output=off  mode=Lower Bit Location + Width  bit1=0  base1=MSB of Input  bit0=10  base0=LSB of Input  dbl_ovrd=off  block_type=slice
  Subsystem1 : Subsystem
  delay_bram_prog_dp : Subsystem  AncestorBlock=casper_library_delays/delay_bram_prog_dp  mask(delay_bram_prog_dp){ram_bits=max_delay_bits-2, bram_latency=2, async=off}
      mask prompts: ram_bits "Max delay (2^?)"; bram_latency "BRAM latency"; async "asynchronous operation"
      mask init:
      | delay_bram_prog_dp_init(gcb, ...
      |     'ram_bits', ram_bits, ...
      |     'bram_latency', bram_latency, ...
      |     'async', async);
  dout : Outport
  wires:
  Subsystem1/1(dout) -> dout/1
  delay_bram_prog_dp/1(dout) -> Subsystem1/1(din)
  Slice1/1 -> Subsystem1/2(delay)
  Slice/1 -> delay_bram_prog_dp/2(delay)
  delay/1 -> Slice/1, Slice1/1
  din/1 -> delay_bram_prog_dp/1(din)

== system snap2_f_200msps_64i_4096c/delay/Subsystem/52 ==
  din : Inport
  delay : Inport  Port=2
  Slice : xbsIndex_r4/Slice  nbits=10  boolean_output=off  mode=Lower Bit Location + Width  bit1=0  base1=MSB of Input  bit0=0  base0=LSB of Input  dbl_ovrd=off  block_type=slice
  Slice1 : xbsIndex_r4/Slice  nbits=2  boolean_output=off  mode=Lower Bit Location + Width  bit1=0  base1=MSB of Input  bit0=10  base0=LSB of Input  dbl_ovrd=off  block_type=slice
  Subsystem1 : Subsystem
  delay_bram_prog_dp : Subsystem  AncestorBlock=casper_library_delays/delay_bram_prog_dp  mask(delay_bram_prog_dp){ram_bits=max_delay_bits-2, bram_latency=2, async=off}
      mask prompts: ram_bits "Max delay (2^?)"; bram_latency "BRAM latency"; async "asynchronous operation"
      mask init:
      | delay_bram_prog_dp_init(gcb, ...
      |     'ram_bits', ram_bits, ...
      |     'bram_latency', bram_latency, ...
      |     'async', async);
  dout : Outport
  wires:
  Subsystem1/1(dout) -> dout/1
  delay_bram_prog_dp/1(dout) -> Subsystem1/1(din)
  Slice1/1 -> Subsystem1/2(delay)
  Slice/1 -> delay_bram_prog_dp/2(delay)
  delay/1 -> Slice/1, Slice1/1
  din/1 -> delay_bram_prog_dp/1(din)

== system snap2_f_200msps_64i_4096c/delay/Subsystem/53 ==
  din : Inport
  delay : Inport  Port=2
  Slice : xbsIndex_r4/Slice  nbits=10  boolean_output=off  mode=Lower Bit Location + Width  bit1=0  base1=MSB of Input  bit0=0  base0=LSB of Input  dbl_ovrd=off  block_type=slice
  Slice1 : xbsIndex_r4/Slice  nbits=2  boolean_output=off  mode=Lower Bit Location + Width  bit1=0  base1=MSB of Input  bit0=10  base0=LSB of Input  dbl_ovrd=off  block_type=slice
  Subsystem1 : Subsystem
  delay_bram_prog_dp : Subsystem  AncestorBlock=casper_library_delays/delay_bram_prog_dp  mask(delay_bram_prog_dp){ram_bits=max_delay_bits-2, bram_latency=2, async=off}
      mask prompts: ram_bits "Max delay (2^?)"; bram_latency "BRAM latency"; async "asynchronous operation"
      mask init:
      | delay_bram_prog_dp_init(gcb, ...
      |     'ram_bits', ram_bits, ...
      |     'bram_latency', bram_latency, ...
      |     'async', async);
  dout : Outport
  wires:
  din/1 -> delay_bram_prog_dp/1(din)
  delay/1 -> Slice1/1, Slice/1
  Slice/1 -> delay_bram_prog_dp/2(delay)
  Slice1/1 -> Subsystem1/2(delay)
  delay_bram_prog_dp/1(dout) -> Subsystem1/1(din)
  Subsystem1/1(dout) -> dout/1

== system snap2_f_200msps_64i_4096c/delay/Subsystem/54 ==
  din : Inport
  delay : Inport  Port=2
  Slice : xbsIndex_r4/Slice  nbits=10  boolean_output=off  mode=Lower Bit Location + Width  bit1=0  base1=MSB of Input  bit0=0  base0=LSB of Input  dbl_ovrd=off  block_type=slice
  Slice1 : xbsIndex_r4/Slice  nbits=2  boolean_output=off  mode=Lower Bit Location + Width  bit1=0  base1=MSB of Input  bit0=10  base0=LSB of Input  dbl_ovrd=off  block_type=slice
  Subsystem1 : Subsystem
  delay_bram_prog_dp : Subsystem  AncestorBlock=casper_library_delays/delay_bram_prog_dp  mask(delay_bram_prog_dp){ram_bits=max_delay_bits-2, bram_latency=2, async=off}
      mask prompts: ram_bits "Max delay (2^?)"; bram_latency "BRAM latency"; async "asynchronous operation"
      mask init:
      | delay_bram_prog_dp_init(gcb, ...
      |     'ram_bits', ram_bits, ...
      |     'bram_latency', bram_latency, ...
      |     'async', async);
  dout : Outport
  wires:
  Subsystem1/1(dout) -> dout/1
  delay_bram_prog_dp/1(dout) -> Subsystem1/1(din)
  Slice1/1 -> Subsystem1/2(delay)
  Slice/1 -> delay_bram_prog_dp/2(delay)
  delay/1 -> Slice/1, Slice1/1
  din/1 -> delay_bram_prog_dp/1(din)

== system snap2_f_200msps_64i_4096c/delay/Subsystem/55 ==
  din : Inport
  delay : Inport  Port=2
  Slice : xbsIndex_r4/Slice  nbits=10  boolean_output=off  mode=Lower Bit Location + Width  bit1=0  base1=MSB of Input  bit0=0  base0=LSB of Input  dbl_ovrd=off  block_type=slice
  Slice1 : xbsIndex_r4/Slice  nbits=2  boolean_output=off  mode=Lower Bit Location + Width  bit1=0  base1=MSB of Input  bit0=10  base0=LSB of Input  dbl_ovrd=off  block_type=slice
  Subsystem1 : Subsystem
  delay_bram_prog_dp : Subsystem  AncestorBlock=casper_library_delays/delay_bram_prog_dp  mask(delay_bram_prog_dp){ram_bits=max_delay_bits-2, bram_latency=2, async=off}
      mask prompts: ram_bits "Max delay (2^?)"; bram_latency "BRAM latency"; async "asynchronous operation"
      mask init:
      | delay_bram_prog_dp_init(gcb, ...
      |     'ram_bits', ram_bits, ...
      |     'bram_latency', bram_latency, ...
      |     'async', async);
  dout : Outport
  wires:
  din/1 -> delay_bram_prog_dp/1(din)
  delay/1 -> Slice1/1, Slice/1
  Slice/1 -> delay_bram_prog_dp/2(delay)
  Slice1/1 -> Subsystem1/2(delay)
  delay_bram_prog_dp/1(dout) -> Subsystem1/1(din)
  Subsystem1/1(dout) -> dout/1

== system snap2_f_200msps_64i_4096c/delay/Subsystem/56 ==
  din : Inport
  delay : Inport  Port=2
  Slice : xbsIndex_r4/Slice  nbits=10  boolean_output=off  mode=Lower Bit Location + Width  bit1=0  base1=MSB of Input  bit0=0  base0=LSB of Input  dbl_ovrd=off  block_type=slice
  Slice1 : xbsIndex_r4/Slice  nbits=2  boolean_output=off  mode=Lower Bit Location + Width  bit1=0  base1=MSB of Input  bit0=10  base0=LSB of Input  dbl_ovrd=off  block_type=slice
  Subsystem1 : Subsystem
  delay_bram_prog_dp : Subsystem  AncestorBlock=casper_library_delays/delay_bram_prog_dp  mask(delay_bram_prog_dp){ram_bits=max_delay_bits-2, bram_latency=2, async=off}
      mask prompts: ram_bits "Max delay (2^?)"; bram_latency "BRAM latency"; async "asynchronous operation"
      mask init:
      | delay_bram_prog_dp_init(gcb, ...
      |     'ram_bits', ram_bits, ...
      |     'bram_latency', bram_latency, ...
      |     'async', async);
  dout : Outport
  wires:
  Subsystem1/1(dout) -> dout/1
  delay_bram_prog_dp/1(dout) -> Subsystem1/1(din)
  Slice1/1 -> Subsystem1/2(delay)
  Slice/1 -> delay_bram_prog_dp/2(delay)
  delay/1 -> Slice/1, Slice1/1
  din/1 -> delay_bram_prog_dp/1(din)
